simulink model "vertical"  (R2025b)
settings: Solver=VariableStepAuto  StartTime=0.0  StopTime=10.0  RelTol=1e-3
values from neighbouring files (symbols this model uses):
  cog_height = Simulink.Parameter    [controller_2022b_saveas.m]
  Fz_stat_FL = Simulink.Parameter    [controller_2022b_saveas.m]
  Fz_stat_FR = Simulink.Parameter    [controller_2022b_saveas.m]
  Fz_stat_RL = Simulink.Parameter    [controller_2022b_saveas.m]
  Fz_stat_RR = Simulink.Parameter    [controller_2022b_saveas.m]
  pitch_inertia = Simulink.Parameter    [controller_2022b_saveas.m]
  pitchAngle = Simulink.Parameter    [controller_2022b_saveas.m]
  pitching_coefficient = Simulink.Parameter    [controller_2022b_saveas.m]
  pitchStiffness = Simulink.Parameter    [controller_2022b_saveas.m]
  rdyn = Simulink.Parameter    [controller_2022b_saveas.m]
  reference_area = Simulink.Parameter    [controller_2022b_saveas.m]
  rho = Simulink.Parameter    [controller_2022b_saveas.m]
  rollStiffness_F = Simulink.Parameter    [controller_2022b_saveas.m]
  rollStiffness_R = Simulink.Parameter    [controller_2022b_saveas.m]
  sprung_mass = Simulink.Parameter    [controller_2022b_saveas.m]
  total_pitchDamping = Simulink.Parameter    [controller_2022b_saveas.m]
  total_pitchStiffness = Simulink.Parameter    [controller_2022b_saveas.m]
  total_rollStiffness = Simulink.Parameter    [controller_2022b_saveas.m]
  trackwidth_F = Simulink.Parameter    [controller_2022b_saveas.m]
  trackwidth_R = Simulink.Parameter    [controller_2022b_saveas.m]
  unsprung_mass = Simulink.Parameter    [controller_2022b_saveas.m]
  wheelbase = Simulink.Parameter    [controller_2022b_saveas.m]
undefined symbols (not defined in the file or in its folder): DiscIntNeverNeededParam
settings Model: Creator=marce  LastModifiedBy=marce

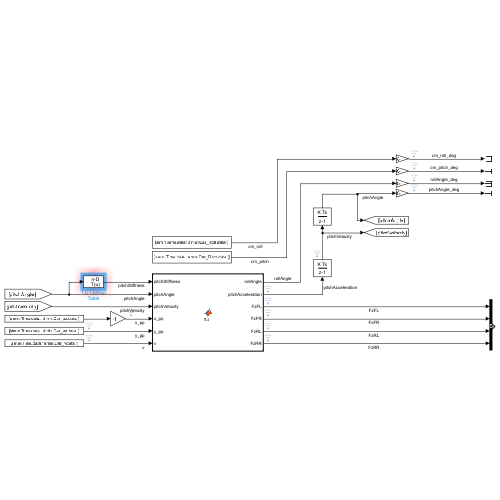
[thumbnail: Simulink's stored preview of the top-level diagram]
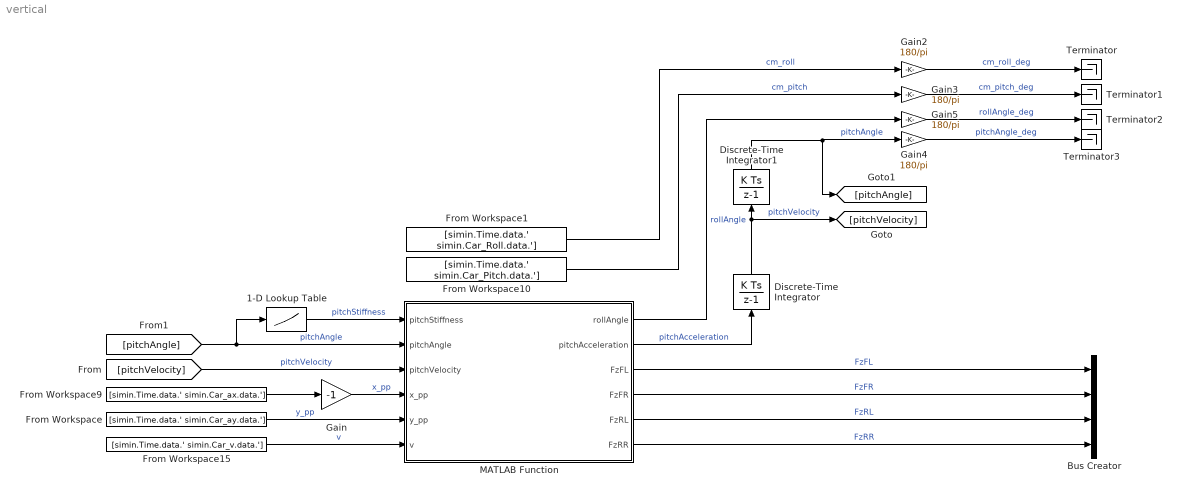
== system vertical ==
  1-D Lookup Table : Lookup_n-D  NumberOfTableDimensions=1  BreakpointsForDimension1=pitchAngle  Table=pitchStiffness  InternalRulePriority=Speed  RndMeth=Simplest
  Bus Creator : BusCreator  Inputs=4
  Discrete-Time Integrator : DiscreteIntegrator  SampleTime=-1  ICPrevOutput=DiscIntNeverNeededParam  ICPrevScaledInput=DiscIntNeverNeededParam
  Discrete-Time Integrator1 : DiscreteIntegrator  InitialCondition=-0.001  SampleTime=-1  ICPrevOutput=DiscIntNeverNeededParam  ICPrevScaledInput=DiscIntNeverNeededParam
  From Workspace : FromWorkspace  VariableName=[simin.Time.data.' simin.Car_ay.data.']  SampleTime=0.01
  From Workspace1 : FromWorkspace  VariableName=[simin.Time.data.' simin.Car_Roll.data.']  SampleTime=0.01
  From Workspace10 : FromWorkspace  VariableName=[simin.Time.data.' simin.Car_Pitch.data.']  SampleTime=0.01
  From Workspace15 : FromWorkspace  VariableName=[simin.Time.data.' simin.Car_v.data.']  SampleTime=0.01
  From Workspace9 : FromWorkspace  VariableName=[simin.Time.data.' simin.Car_ax.data.']  SampleTime=0.01
  Gain : Gain  Gain=-1
  Gain{2..5} (4 alike) : Gain  Gain=180/pi
  MATLAB Function : MATLAB Function  TreatAsAtomicUnit=on
  Terminator{,1..3} (4 alike) : Terminator
  wires:
  MATLAB Function/6(FzRR) -> Bus Creator/4  "FzRR"
  1-D Lookup Table/1 -> MATLAB Function/1(pitchStiffness)  "pitchStiffness"
  Gain/1 -> MATLAB Function/4(x_pp)  "x_pp"
  Discrete-Time Integrator1/1 -> Gain4/1, [pitchAngle]  "pitchAngle"
  From Workspace15/1 -> MATLAB Function/6(v)  "v"
  From Workspace1/1 -> Gain2/1  "cm_roll"
  MATLAB Function/4(FzFR) -> Bus Creator/2  "FzFR"
  From Workspace/1 -> MATLAB Function/5(y_pp)  "y_pp"
  From Workspace9/1 -> Gain/1
  MATLAB Function/3(FzFL) -> Bus Creator/1  "FzFL"
  From Workspace10/1 -> Gain3/1  "cm_pitch"
  Gain5/1 -> Terminator2/1  "rollAngle_deg"
  Gain4/1 -> Terminator3/1  "pitchAngle_deg"
  MATLAB Function/5(FzRL) -> Bus Creator/3  "FzRL"
  [pitchAngle] -> 1-D Lookup Table/1, MATLAB Function/2(pitchAngle)  "pitchAngle"
  Discrete-Time Integrator/1 -> [pitchVelocity], Discrete-Time Integrator1/1  "pitchVelocity"
  Gain2/1 -> Terminator/1  "cm_roll_deg"
  [pitchVelocity] -> MATLAB Function/3(pitchVelocity)  "pitchVelocity"
  MATLAB Function/2(pitchAcceleration) -> Discrete-Time Integrator/1  "pitchAcceleration"
  MATLAB Function/1(rollAngle) -> Gain5/1  "rollAngle"
  Gain3/1 -> Terminator1/1  "cm_pitch_deg"

== matlab function vertical/MATLAB Function ==
  data: pitchStiffness input; pitchAngle input; pitchVelocity input; x_pp input; rollAngle output; pitchAcceleration output; y_pp input; v input; cog_height parameter; sprung_mass parameter; FzFL output; rollStiffness_F parameter; rollStiffness_R parameter; total_rollStiffness parameter; trackwidth_F parameter; trackwidth_R parameter; Fz_stat_FL parameter; Fz_stat_FR parameter; Fz_stat_RL parameter; Fz_stat_RR parameter; FzFR output; FzRL output; FzRR output; wheelbase parameter; total_pitchStiffness parameter; rdyn parameter; unsprung_mass parameter; pitch_inertia parameter; total_pitchDamping parameter; reference_area parameter; pitching_coefficient parameter; rho parameter
function [rollAngle,pitchAcceleration,FzFL,FzFR,FzRL,FzRR]  = fcn(pitchStiffness,pitchAngle,pitchVelocity,x_pp, y_pp,v, cog_height, sprung_mass,rollStiffness_F,rollStiffness_R,total_rollStiffness,trackwidth_F, trackwidth_R, Fz_stat_FL, Fz_stat_FR, Fz_stat_RL, Fz_stat_RR, wheelbase, total_pitchStiffness, rdyn, unsprung_mass, pitch_inertia, total_pitchDamping, reference_area, pitching_coefficient, rho)

rollTorque = sprung_mass .* y_pp .* cog_height;
rollAngle = rollTorque ./ (total_rollStiffness);

dFz_roll_FL = (rollAngle .* rollStiffness_F - rdyn .* unsprung_mass .* y_pp) ./ trackwidth_F;
dFz_roll_FR = (rollAngle .* rollStiffness_F - rdyn .* unsprung_mass .* y_pp) ./ trackwidth_F;
dFz_roll_RL = (rollAngle .* rollStiffness_R - rdyn .* unsprung_mass .* y_pp) ./ trackwidth_R;
dFz_roll_RR = (rollAngle .* rollStiffness_R - rdyn .* unsprung_mass .* y_pp) ./ trackwidth_R;
           
pitchTorque = sprung_mass .* x_pp .* cog_height - rho ./2 .* pitching_coefficient .* wheelbase .* reference_area .* v^2;
% pitchStiffness = 3.825903e+09 * pitchAngle^3 + -1.854731e+09 * pitchAngle^2 + 1.728035e+08 * pitchAngle + -1.759672e+06;
% pitchStiffness = min(max(pitchStiffness, 290e3), 626e3);
pitchAcceleration = (pitchTorque - total_pitchDamping .* pitchVelocity - pitchStiffness .* pitchAngle) ./ pitch_inertia;

dFz_pitch_FL = (pitchStiffness ./ 2 .* pitchAngle + total_pitchDamping ./ 2 .* pitchVelocity - pitch_inertia ./4 .* pitchAcceleration) ./ wheelbase;
dFz_pitch_FR = (pitchStiffness ./ 2 .* pitchAngle + total_pitchDamping ./ 2 .* pitchVelocity - pitch_inertia ./4 .* pitchAcceleration) ./ wheelbase;
dFz_pitch_RL = (pitchStiffness ./ 2 .* pitchAngle + total_pitchDamping ./ 2 .* pitchVelocity - pitch_inertia ./4 .* pitchAcceleration) ./ wheelbase;
dFz_pitch_RR = (pitchStiffness ./ 2 .* pitchAngle + total_pitchDamping ./ 2 .* pitchVelocity - pitch_inertia ./4 .* pitchAcceleration) ./ wheelbase;

FzFL = Fz_stat_FL + dFz_roll_FL + dFz_pitch_FL;
FzFR = Fz_stat_FR - dFz_roll_FR + dFz_pitch_FR;
FzRL = Fz_stat_RL + dFz_roll_RL - dFz_pitch_RL;
FzRR = Fz_stat_RR - dFz_roll_RR - dFz_pitch_RR;
